simulink model "mech_gimbal_transform"  (Simulink 7.1)
settings: Solver=ode45  StartTime=0.0  StopTime=10  MaxStep=.001  RelTol=1e-3
libraries: mblibv1 x11
Description:
  | Gimbal Transform
  | 
  | This mode demonstrates the relationship between the motion of
  | each of the primitives of a Gimbal joint and the rate and acceleration
  | of the body it is connected to.
settings Model: Creator=The MathWorks Inc.
settings DataIOCC: LimitDataPoints=off  OutputOption=SpecifiedOutputTimes  OutputTimes=[0:.010:2]
settings DebuggingCC: SaveWithParameterizedLinksMsg=none  SignalResolutionControl=TryResolveAllWithWarning  MultiTaskDSMMsg=warning  MultiTaskCondExecSysMsg=none  UnconnectedLineMsg=none
settings RTWCC: IncludeERTFirstTime=on
settings GRTTargetCC: TargetFcnLib=ansi_tfl_tmw.mat

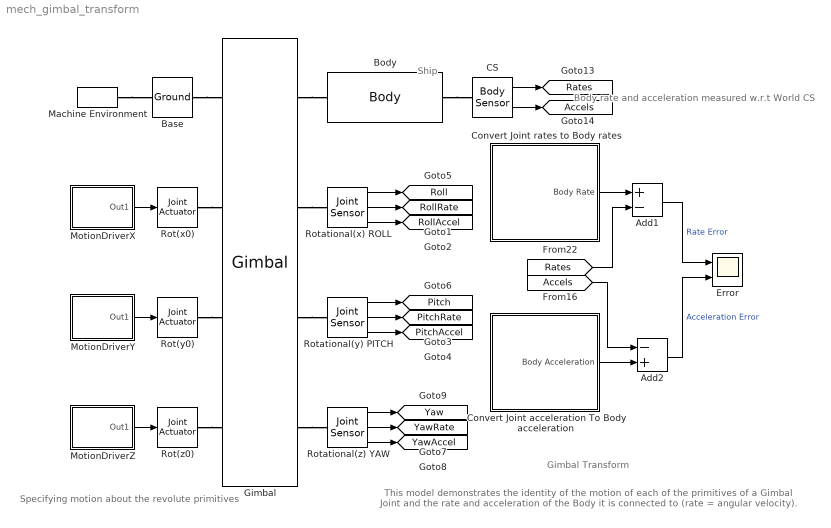
== system mech_gimbal_transform ==
  note: Body rate and acceleration
      | measured w.r.t World CS
  note: Specifying motion about
      | the revolute primitives
  note: Ship
  note: Gimbal Transform
  note: This model demonstrates the identity of the motion of
      | each of the primitives of a Gimbal Joint and the rate and acceleration
      | of the Body it is connected to (rate = angular velocity).
  Add1 : Sum  Inputs=+-  OutDataType=sfix(16)  OutScaling=2^-10
  Add2 : Sum  Inputs=-+  OutDataType=sfix(16)  OutScaling=2^-10
  Base : mblibv1/Bodies/Ground  DialogController=MECH.DynMechDlgSource  SystemSampleTime=-1  LeftPortType=env  RightPortType=workingframe  PhysicalDomain=Mechanical  DialogClass=GroundBlock  CoordPosition=[0 0 0]  CoordPositionUnits=m  StateVectorMgrId=-1  MachineId=[0 0]  ShowEnvPort=on
  Body : mblibv1/Bodies/Body  DialogController=MECH.DynMechDlgSource  PhysicalDomain=mechanical  SubClassName=Unknown  LeftPortType=workingframe  RightPortType=workingframe  LConnTagsString=CS1  RConnTagsString=CS8  DialogClass=MechanicalBodyBlock  Mass=1  MassUnits=kg  InertiaUnits=kg*m^2  Inertia=[0.06 0 0;0 0.7 0;0 0 0.75]*0.25  Shape=Cylinder  ShapeDims=[1 1]  ShapeUnits=m  ShapeUse=false  Density=1  DensityUnits=kg/m^3  DensityUse=false  GraphicsMode=1  BodyColor=[0.5 0.5 0.5]  GraphicsObj=[]  AttachedToCS=1  CG=Right$CG$[0 0 0]$WORLD$WORLD$m$[0 0 0]$Euler X-Y-Z$deg$WORLD$false  WorkingFrames="Left$CS1$[0 0 0]$WORLD$WORLD$m$[0 0 0]$Euler X-Y-Z$deg$WORLD$true#Right$CS8$[0 0 0]$WORLD$WORLD$m$[0 0 0]$Euler X-Y-Z$deg$WORLD$true#Left$CS2$[-87.81 -10 0]$WORLD$WORLD$cm$[0 0 0]$Euler X-Y-Z$deg$WORLD$false#Left$CS5$[-87.81 -8 -10]$WORLD$WORLD$cm$[0 0 0]$Euler X-Y-Z$deg$WORLD$false#Left$CS3$[-87.81  10 0]$WORLD$WORLD$cm$[0 0 0]$Euler X-Y-Z$deg$WORLD$false#Left$CS6$[-87.81 8 -10]$WORLD$WORLD$cm$[0 0 0]$Euler X-Y-Z$deg$WORLD$false#Right$CS4$[94.99  0 0]$WORLD$WORLD$cm$[0 0 0]$Euler X-Y-Z$deg$WORLD$false#Left$CS7$[80.0  0 -10]$WORLD$WORLD$cm$[0 0 0]$Euler X-Y-Z$deg$WORLD$false"  CGPos=[0 0 0]  CGRot=[0 0 0]  CS0Pos=[]  CS0Rot=[]  CS1Pos=[0 0 0]  CS1Rot=[0 0 0]  CS2Pos=[-87.81 -10 0]  CS2Rot=[0 0 0]  CS3Pos="[-87.81  10 0]"  CS3Rot=[0 0 0]  CS4Pos="[94.99  0 0]"  CS4Rot=[0 0 0]  CS5Pos=[-87.81 -8 -10]  CS5Rot=[0 0 0]  CS6Pos=[-87.81 8 -10]  CS6Rot=[0 0 0]  CS7Pos="[80.0  0 -10]"  CS7Rot=[0 0 0]  CS8Pos=[0 0 0]  CS8Rot=[0 0 0]  CS9Pos=[]  CS9Rot=[]  CS10Pos=[]  CS10Rot=[]  CS11Pos=[]  CS11Rot=[]  CS12Pos=[]  CS12Rot=[]  CS13Pos=[]  CS13Rot=[]  CS14Pos=[]  CS14Rot=[]  CS15Pos=[]  CS15Rot=[]  CS16Pos=[]  CS16Rot=[]  CS17Pos=[]  CS17Rot=[]  CS18Pos=[]  CS18Rot=[]  CS19Pos=[]  CS19Rot=[]  CS20Pos=[]  CS20Rot=[]
  CS : mblibv1/Sensors &  Actuators/Body Sensor  DialogController=MECH.DynMechDlgSource  SystemSampleTime=-1  PhysicalDomain=Mechanical  PortType=blob  Muxed=off  Pose=off  Angle=on  AngleUnits=deg  ArcVelocity=on  ArcVelocityUnits=rad/s  ArcAcceleration=on  ArcAccelerationUnits=rad/s^2  CoordPosition=off  CoordPositionUnits=m  Velocity=off  VelocityUnits=m/s  Acceleration=off  AccelerationUnits=m/s^2  Quaternion=on  QuaternionDT=off  QuaternionDDT=off  QuaternionUnits=off  OutputVector=[ 3 3 ]  ActiveIO=on  Width=6  DialogClass=MechanicalSensorBlock  ReferenceFrame=Absolute (World)
  Convert Joint acceleration To Body acceleration : Subsystem
  Convert Joint rates to Body rates : Subsystem
  Error : Scope  NumInputPorts=2
      settings: TimeRange=10  YMin=-1~-8.000000000000001e-018  YMax=1~8.000000000000001e-018
  Gimbal : mblibv1/Joints/Gimbal  DialogController=MECH.DynMechDlgSource  PhysicalDomain=mechanical  SubClassName=Unknown  LeftPortType=blob  RightPortType=blob  LConnTagsString=__newl0|SA1|SA2|SA3  RConnTagsString=__newr0|SA1|SA2|SA3  NumSAPorts=6  CutJoint=off  MarkAsCut=off  Primitives=revolute_revolute_revolute  PrimitiveProps=R1$WORLD$[1 0 0]$revolute#R2$WORLD$[0 1 0]$revolute#R3$WORLD$[0 0 1]$revolute  DialogClass=JointBlock  R1Axis=[1 0 0]  R2Axis=[0 1 0]  R3Axis=[0 0 1]
  Machine Environment : mblibv1/Bodies/Machine Environment  Tag=Factory ground  DialogController=MECH.DialogSource  SystemSampleTime=-1  PortType=env  PhysicalDomain=Mechanical  DialogTemplateClass=MECH.MachineEnvironment  SyncWhenCopied=off  Gravity=[0 0 0]  GravityUnits=m/s^2  GravityAsSignal=off  Dimensionality=3D Only  AnalysisType=Forward dynamics  LinearAssemblyTolerance=1e-6  LinearAssemblyToleranceUnits=m  AngularAssemblyTolerance=1e-4  AngularAssemblyToleranceUnits=rad  ConstraintSolverType=Stabilizing  ConstraintRelTolerance=1e-4  ConstraintAbsTolerance=1e-4  UseRobustSingularityHandling=on  RedundancyAnalysisToleranceType=Automatically select tolerance  RedundancyAnalysisTolerance=1e-14  StatePerturbationType=Adaptive  PerturbationSize=1e-5  VisualizeMachine=on
  MotionDriverX : Subsystem
  MotionDriverY : Subsystem
  MotionDriverZ : Subsystem
  Rot(x0) : mblibv1/Sensors &  Actuators/Joint Actuator  DialogController=MECH.DynMechDlgSource  SystemSampleTime=-1  PhysicalDomain=Mechanical  PortType=blob  ActuationStyle=Motion  AngleUnits=deg  ArcVelocityUnits=deg/s  ArcAccelerationUnits=deg/s^2  CoordPositionUnits=m  VelocityUnits=m/s  AccelerationUnits=m/s^2  ForceUnits=N  TorqueUnits=N-m  ActiveIO=on  Width=3  DialogClass=MechanicalActuatorBlock  Primitive=R1  ReferenceFrame=Absolute (INERTIAL)
  Rot(y0) : mblibv1/Sensors &  Actuators/Joint Actuator  DialogController=MECH.DynMechDlgSource  SystemSampleTime=-1  PhysicalDomain=Mechanical  PortType=blob  ActuationStyle=Motion  AngleUnits=deg  ArcVelocityUnits=deg/s  ArcAccelerationUnits=deg/s^2  CoordPositionUnits=m  VelocityUnits=m/s  AccelerationUnits=m/s^2  ForceUnits=N  TorqueUnits=N-m  ActiveIO=on  Width=3  DialogClass=MechanicalActuatorBlock  Primitive=R2  ReferenceFrame=Absolute (INERTIAL)
  Rot(z0) : mblibv1/Sensors &  Actuators/Joint Actuator  DialogController=MECH.DynMechDlgSource  SystemSampleTime=-1  PhysicalDomain=Mechanical  PortType=blob  ActuationStyle=Motion  AngleUnits=deg  ArcVelocityUnits=deg/s  ArcAccelerationUnits=deg/s^2  CoordPositionUnits=m  VelocityUnits=m/s  AccelerationUnits=m/s^2  ForceUnits=N  TorqueUnits=N-m  ActiveIO=on  Width=3  DialogClass=MechanicalActuatorBlock  Primitive=R3  ReferenceFrame=Absolute (INERTIAL)
  Rotational(x) ROLL : mblibv1/Sensors &  Actuators/Joint Sensor  DialogController=MECH.DynMechDlgSource  SystemSampleTime=-1  PhysicalDomain=Mechanical  PortType=blob  Muxed=off  Pose=off  Angle=on  AngleUnits=rad  ArcVelocity=on  ArcVelocityUnits=rad/s  ArcAcceleration=on  ArcAccelerationUnits=rad/s^2  CoordPosition=on  CoordPositionUnits=m  Velocity=off  VelocityUnits=m/s  Acceleration=off  AccelerationUnits=m/s^2  Quaternion=on  QuaternionDT=off  QuaternionDDT=off  QuaternionUnits=off  OutputVector=[ 1 1 1 ]  ActiveIO=on  Width=3  DialogClass=MechanicalSensorBlock  Primitive=R1  Force=off  ForceUnits=N  Torque=off  TorqueUnits=N-m  ReferenceFrame=Absolute (INERTIAL)  ReactionSensedSide=Base  ReactionReferenceFrame=Absolute (World)  ReactionForce=off  ReactionForceUnits=N  ReactionMoment=off  ReactionMomentUnits=N-m
  Rotational(y) PITCH : mblibv1/Sensors &  Actuators/Joint Sensor  DialogController=MECH.DynMechDlgSource  SystemSampleTime=-1  PhysicalDomain=Mechanical  PortType=blob  Muxed=off  Pose=off  Angle=on  AngleUnits=rad  ArcVelocity=on  ArcVelocityUnits=rad/s  ArcAcceleration=on  ArcAccelerationUnits=rad/s^2  CoordPosition=on  CoordPositionUnits=m  Velocity=off  VelocityUnits=m/s  Acceleration=off  AccelerationUnits=m/s^2  Quaternion=on  QuaternionDT=off  QuaternionDDT=off  QuaternionUnits=off  OutputVector=[ 1 1 1 ]  ActiveIO=on  Width=3  DialogClass=MechanicalSensorBlock  Primitive=R2  Force=off  ForceUnits=N  Torque=off  TorqueUnits=N-m  ReferenceFrame=Absolute (INERTIAL)  ReactionSensedSide=Base  ReactionReferenceFrame=Absolute (World)  ReactionForce=off  ReactionForceUnits=N  ReactionMoment=off  ReactionMomentUnits=N-m
  Rotational(z) YAW : mblibv1/Sensors &  Actuators/Joint Sensor  DialogController=MECH.DynMechDlgSource  SystemSampleTime=-1  PhysicalDomain=Mechanical  PortType=blob  Muxed=off  Pose=off  Angle=on  AngleUnits=rad  ArcVelocity=on  ArcVelocityUnits=rad/s  ArcAcceleration=on  ArcAccelerationUnits=rad/s^2  CoordPosition=on  CoordPositionUnits=m  Velocity=off  VelocityUnits=m/s  Acceleration=off  AccelerationUnits=m/s^2  Quaternion=on  QuaternionDT=off  QuaternionDDT=off  QuaternionUnits=off  OutputVector=[ 1 1 1 ]  ActiveIO=on  Width=3  DialogClass=MechanicalSensorBlock  Primitive=R3  Force=off  ForceUnits=N  Torque=off  TorqueUnits=N-m  ReferenceFrame=Absolute (INERTIAL)  ReactionSensedSide=Base  ReactionReferenceFrame=Absolute (World)  ReactionForce=off  ReactionForceUnits=N  ReactionMoment=off  ReactionMomentUnits=N-m
  tag scope: Accels=global, Pitch=global, PitchAccel=global, PitchRate=global, Rates=global, Roll=global, RollAccel=global, RollRate=global, Yaw=global, YawAccel=global, YawRate=global
  wires:
  Rotational(x) ROLL/1 -> [Roll]
  Rotational(y) PITCH/1 -> [Pitch]
  MotionDriverX/1(Out1) -> Rot(x0)/1
  CS/1 -> [Rates]
  CS/2 -> [Accels]
  MotionDriverY/1(Out1) -> Rot(y0)/1
  Rotational(x) ROLL/2 -> [RollRate]
  Rotational(x) ROLL/3 -> [RollAccel]
  Rotational(y) PITCH/2 -> [PitchRate]
  Rotational(y) PITCH/3 -> [PitchAccel]
  Rotational(z) YAW/1 -> [Yaw]
  Rotational(z) YAW/2 -> [YawRate]
  Rotational(z) YAW/3 -> [YawAccel]
  MotionDriverZ/1(Out1) -> Rot(z0)/1
  Convert Joint rates to Body rates/1(Body Rate) -> Add1/1
  [Rates] -> Add1/2
  Add1/1 -> Error/1  "Rate Error"
  Add2/1 -> Error/2  "Acceleration Error"
  [Accels] -> Add2/1
  Convert Joint acceleration To Body acceleration/1(Body Acceleration) -> Add2/2
  connections:
  Machine Environment/RConn1 -- Base/LConn1
  Rot(y0)/RConn1 -- Gimbal/LConn3
  Rot(x0)/RConn1 -- Gimbal/LConn2
  Gimbal/RConn2 -- Rotational(x) ROLL/LConn1
  Gimbal/RConn3 -- Rotational(y) PITCH/LConn1
  Gimbal/RConn4 -- Rotational(z) YAW/LConn1
  Base/RConn1 -- Gimbal/LConn1
  Gimbal/RConn1 -- Body/LConn1
  Rot(z0)/RConn1 -- Gimbal/LConn4
  Body/RConn1 -- CS/LConn1

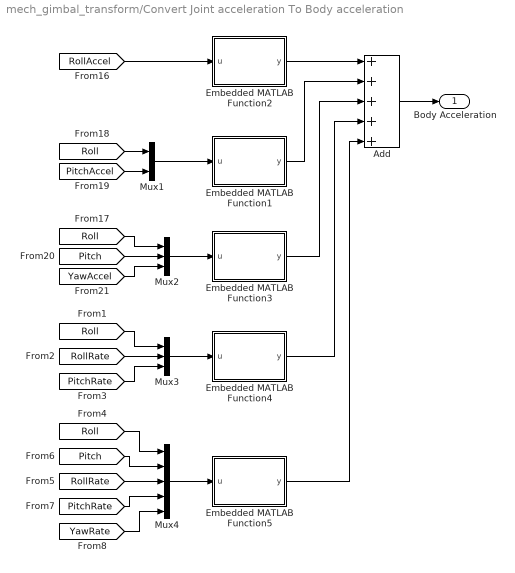
== system mech_gimbal_transform/Convert Joint acceleration To Body acceleration ==
  Add : Sum  Inputs=+++++  OutDataType=sfix(16)  OutScaling=2^-10
  Embedded MATLAB Function1 : Stateflow chart
  Embedded MATLAB Function2 : Stateflow chart
  Embedded MATLAB Function3 : Stateflow chart
  Embedded MATLAB Function4 : Stateflow chart
  Embedded MATLAB Function5 : Stateflow chart
  Mux1 : Mux  Inputs=2
  Mux2 : Mux  Inputs=3
  Mux3 : Mux  Inputs=3
  Mux4 : Mux  Inputs=5
  Body Acceleration : Outport  OutDataType=sfix(16)  OutScaling=2^0
  wires:
  Add/1 -> Body Acceleration/1
  Embedded MATLAB Function3/1(y) -> Add/3
  Embedded MATLAB Function1/1(y) -> Add/2
  Embedded MATLAB Function2/1(y) -> Add/1
  [YawAccel] -> Mux2/3
  Mux2/1 -> Embedded MATLAB Function3/1(u)
  [Pitch] -> Mux2/2
  [RollAccel] -> Embedded MATLAB Function2/1(u)
  Mux1/1 -> Embedded MATLAB Function1/1(u)
  [PitchAccel] -> Mux1/2
  [Roll] -> Mux1/1
  [Roll] -> Mux3/1
  [RollRate] -> Mux3/2
  [PitchRate] -> Mux3/3
  Mux3/1 -> Embedded MATLAB Function4/1(u)
  [Roll] -> Mux4/1
  [PitchRate] -> Mux4/4
  [YawRate] -> Mux4/5
  Mux4/1 -> Embedded MATLAB Function5/1(u)
  [Pitch] -> Mux4/2
  [RollRate] -> Mux4/3
  Embedded MATLAB Function4/1(y) -> Add/4
  Embedded MATLAB Function5/1(y) -> Add/5
  [Roll] -> Mux2/1

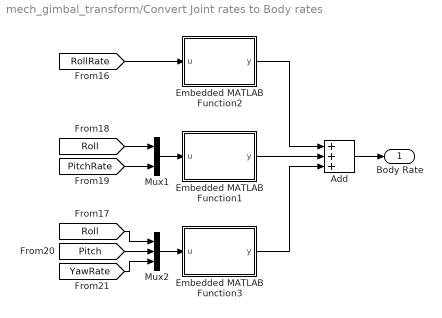
== system mech_gimbal_transform/Convert Joint rates to Body rates ==
  Add : Sum  Inputs=+++  OutDataType=sfix(16)  OutScaling=2^-10
  Embedded MATLAB Function1 : Stateflow chart
  Embedded MATLAB Function2 : Stateflow chart
  Embedded MATLAB Function3 : Stateflow chart
  Mux1 : Mux  Inputs=2
  Mux2 : Mux  Inputs=3
  Body Rate : Outport  OutDataType=sfix(16)  OutScaling=2^0
  wires:
  [Roll] -> Mux1/1
  [PitchRate] -> Mux1/2
  Mux1/1 -> Embedded MATLAB Function1/1(u)
  [RollRate] -> Embedded MATLAB Function2/1(u)
  [Pitch] -> Mux2/2
  Mux2/1 -> Embedded MATLAB Function3/1(u)
  [YawRate] -> Mux2/3
  Embedded MATLAB Function2/1(y) -> Add/1
  Embedded MATLAB Function1/1(y) -> Add/2
  Embedded MATLAB Function3/1(y) -> Add/3
  Add/1 -> Body Rate/1
  [Roll] -> Mux2/1

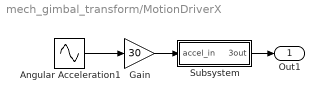
== system mech_gimbal_transform/MotionDriverX ==
  Angular Acceleration1 : Sin  Amplitude=.1  SampleTime=0
  Gain : Gain  Gain=30  ParameterDataType=sfix(16)  ParameterScaling=2^0  OutDataType=sfix(16)  OutScaling=2^0  SaturateOnIntegerOverflow=on  OutDataTypeStr=Inherit: Same as input  ParamDataTypeStr=Inherit: Same as input
  Subsystem : Subsystem
  Out1 : Outport  OutDataType=sfix(16)  OutScaling=2^0
  wires:
  Angular Acceleration1/1 -> Gain/1
  Gain/1 -> Subsystem/1(accel_in)
  Subsystem/1(3out) -> Out1/1

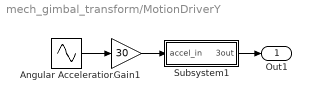
== system mech_gimbal_transform/MotionDriverY ==
  Angular Acceleration : Sin  Amplitude=.1  Phase=30  SampleTime=0
  Gain1 : Gain  Gain=30  ParameterDataType=sfix(16)  ParameterScaling=2^0  OutDataType=sfix(16)  OutScaling=2^0  SaturateOnIntegerOverflow=on  OutDataTypeStr=Inherit: Same as input  ParamDataTypeStr=Inherit: Same as input
  Subsystem1 : Subsystem
  Out1 : Outport  OutDataType=sfix(16)  OutScaling=2^0
  wires:
  Angular Acceleration/1 -> Gain1/1
  Gain1/1 -> Subsystem1/1(accel_in)
  Subsystem1/1(3out) -> Out1/1

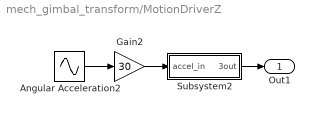
== system mech_gimbal_transform/MotionDriverZ ==
  Angular Acceleration2 : Sin  Amplitude=.1  SampleTime=0
  Gain2 : Gain  Gain=30  ParameterDataType=sfix(16)  ParameterScaling=2^0  OutDataType=sfix(16)  OutScaling=2^0  SaturateOnIntegerOverflow=on  OutDataTypeStr=Inherit: Same as input  ParamDataTypeStr=Inherit: Same as input
  Subsystem2 : Subsystem
  Out1 : Outport  OutDataType=sfix(16)  OutScaling=2^0
  wires:
  Gain2/1 -> Subsystem2/1(accel_in)
  Angular Acceleration2/1 -> Gain2/1
  Subsystem2/1(3out) -> Out1/1

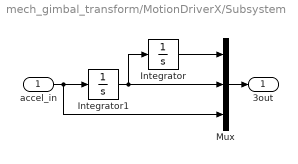
== system mech_gimbal_transform/MotionDriverX/Subsystem ==
  accel_in : Inport  OutDataType=sfix(16)  OutScaling=2^0
  Integrator : Integrator
  Integrator1 : Integrator
  Mux : Mux  Inputs=3
  3out : Outport  OutDataType=sfix(16)  OutScaling=2^0
  wires:
  accel_in/1 -> Integrator1/1, Mux/3
  Integrator1/1 -> Integrator/1, Mux/2
  Integrator/1 -> Mux/1
  Mux/1 -> 3out/1

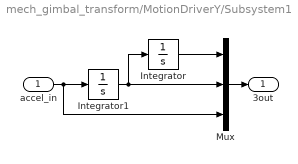
== system mech_gimbal_transform/MotionDriverY/Subsystem1 ==
  accel_in : Inport  OutDataType=sfix(16)  OutScaling=2^0
  Integrator : Integrator
  Integrator1 : Integrator
  Mux : Mux  Inputs=3
  3out : Outport  OutDataType=sfix(16)  OutScaling=2^0
  wires:
  Mux/1 -> 3out/1
  Integrator/1 -> Mux/1
  Integrator1/1 -> Mux/2, Integrator/1
  accel_in/1 -> Mux/3, Integrator1/1

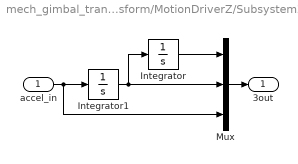
== system mech_gimbal_transform/MotionDriverZ/Subsystem2 ==
  accel_in : Inport  OutDataType=sfix(16)  OutScaling=2^0
  Integrator : Integrator
  Integrator1 : Integrator
  Mux : Mux  Inputs=3
  3out : Outport  OutDataType=sfix(16)  OutScaling=2^0
  wires:
  Mux/1 -> 3out/1
  Integrator/1 -> Mux/1
  Integrator1/1 -> Mux/2, Integrator/1
  accel_in/1 -> Mux/3, Integrator1/1

== matlab function Convert Joint rates to Body rates/Embedded MATLAB Function1 ==
  data: u input double; y output double
function y = fcn(u)
% This block supports an embeddable subset of the MATLAB language.
% See the help menu for details. 

Rx = [1 0 0; 0 cos(u(1)) -sin(u(1)); 0 sin(u(1)) cos(u(1))];
U = [0 u(2) 0]';

y = Rx*U;

== matlab function Convert Joint rates to Body rates/Embedded MATLAB Function2 ==
  data: u input double; y output double
function y = fcn(u)
% This block supports an embeddable subset of the MATLAB language.
% See the help menu for details. 

y = [u 0 0]';

== matlab function Convert Joint rates to Body rates/Embedded MATLAB Function3 ==
  data: u input double; y output double
function y = fcn(u)
% This block supports an embeddable subset of the MATLAB language.
% See the help menu for details. 

Rx = [1 0 0; 0 cos(u(1)) -sin(u(1)); 0 sin(u(1)) cos(u(1))];
Ry = [cos(u(2)) 0 sin(u(2)); 0 1 0; -sin(u(2)) 0 cos(u(2))];
R = Rx*Ry;
U = [0 0 u(3)]';

y = R*U;

== matlab function Convert Joint acceleration To Body acceleration/Embedded MATLAB Function1 ==
  data: u input double; y output double
function y = fcn(u)
% This block supports an embeddable subset of the MATLAB language.
% See the help menu for details. 

Rx = [1 0 0; 0 cos(u(1)) -sin(u(1)); 0 sin(u(1)) cos(u(1))];
U = [0 u(2) 0]';

y = Rx*U;

== matlab function Convert Joint acceleration To Body acceleration/Embedded MATLAB Function2 ==
  data: u input double; y output double
function y = fcn(u)
% This block supports an embeddable subset of the MATLAB language.
% See the help menu for details. 

y = [u 0 0]';

== matlab function Convert Joint acceleration To Body acceleration/Embedded MATLAB Function3 ==
  data: u input double; y output double
function y = fcn(u)
% This block supports an embeddable subset of the MATLAB language.
% See the help menu for details. 

Rx = [1 0 0; 0 cos(u(1)) -sin(u(1)); 0 sin(u(1)) cos(u(1))];
Ry = [cos(u(2)) 0 sin(u(2)); 0 1 0; -sin(u(2)) 0 cos(u(2))];
R = Rx*Ry;
U = [0 0 u(3)]';

y = R*U;

== matlab function Convert Joint acceleration To Body acceleration/Embedded MATLAB Function4 ==
  data: u input double; y output double
function y = fcn(u)
% This block supports an embeddable subset of the MATLAB language.
% See the help menu for details. 

Rx_d = [0 0 0; 0 -sin(u(1)) -cos(u(1)); 0 cos(u(1)) -sin(u(1))]*u(2);
U = [0 u(3) 0]';

y = Rx_d*U;

== matlab function Convert Joint acceleration To Body acceleration/Embedded MATLAB Function5 ==
  data: u input double; y output double
function y = fcn(u)
% This block supports an embeddable subset of the MATLAB language.
% See the help menu for details. 

Rx = [1 0 0; 0 cos(u(1)) -sin(u(1)); 0 sin(u(1)) cos(u(1))];
Ry = [cos(u(2)) 0 sin(u(2)); 0 1 0; -sin(u(2)) 0 cos(u(2))];
Rx_d = [0 0 0; 0 -sin(u(1)) -cos(u(1)); 0 cos(u(1)) -sin(u(1))]*u(3);
Ry_d = [-sin(u(2)) 0 cos(u(2)); 0 0 0; -cos(u(2)) 0 -sin(u(2))]*u(4);
U = [0 0 u(5)]';

y = [Rx_d*Ry + Rx*Ry_d]*U;
